simulink model "TP_Avion_Eleve_a"  (R2018a)
settings: Solver=VariableStepAuto  StartTime=0.0  StopTime=400  RelTol=1e-3
libraries: slctrlblks x1, simulink x1
settings Model: Creator=xpess  LastModifiedBy=xpess
settings DebuggingCC: LibraryContextMissingDiagnostic=warning
settings SFSimCC: SimUseLocalCustomCode=on
settings RTWCC: RTWUseLocalCustomCode=on

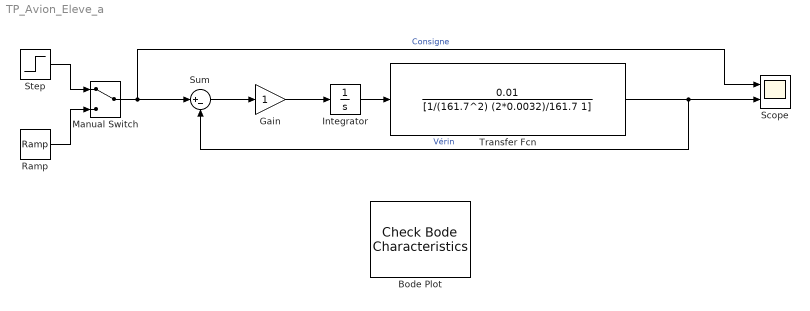
== system TP_Avion_Eleve_a ==
  Bode Plot : slctrlblks/Model Verification/Check Bode  Characteristics  InstantiateOnLoad=on  SaveOperatingPoints=off  LinearizationIOs={'/Sum', 1, 'in', 'on', '';'/Transfer Fcn', 1, 'out', 'on', ''}  LinearizeAt=SnapshotTimes  SnapshotTimes=[0]  TriggerType=rising  SampleTime=auto  RateConversionMethod=zoh  PreWarpFreq=10  UseExactDelayModel=off  UseFullBlockNameLabels=off  UseBusSignalLabels=off  enabled=on  stopWhenAssertionFail=off  export=off  ViewDlgPos=[100 200 510 390]  OpenViewOnLoad=off  LaunchViewOnOpen=on  FrequencyUnits=rad/s  MagnitudeUnits=dB  PhaseUnits=deg  TimeUnits=seconds  EnableUpperBound=off  UpperBoundFrequencies=[]  UpperBoundMagnitudes=[]  EnableLowerBound=off  LowerBoundFrequencies=[]  LowerBoundMagnitudes=[]
      settings: SourceProductName=Simulink Control Design
  Gain : Gain
  Integrator : Integrator
  Manual Switch : ManualSwitch
  Ramp : simulink/Sources/Ramp  slope=1  start=0  InitialOutput=0
  Scope : Scope  NumInputPorts=2
  Step : Step  Time=0  SampleTime=0
  Sum : Sum  Inputs=|+-
  Transfer Fcn : TransferFcn  Numerator=[0.01]  Denominator=[1/(161.7^2) (2*0.0032)/161.7 1]
  wires:
  Step/1 -> Manual Switch/1
  Sum/1 -> Gain/1
  Transfer Fcn/1 -> Scope/2, Sum/2  "Vérin"
  Integrator/1 -> Transfer Fcn/1
  Gain/1 -> Integrator/1
  Ramp/1 -> Manual Switch/2
  Manual Switch/1 -> Scope/1, Sum/1  "Consigne"
